simulink model "grua_portuaria"  (R2021a)
settings: Solver=VariableStepAuto  StartTime=0.0  StopTime=2  RelTol=1e-3
values from neighbouring files (symbols this model uses):
  b_cx = 1*10^6    (= 1000000)    [parametros.m]
  b_cy = 1*10^7    (= 10000000)    [parametros.m]
  b_eq = (b_td+b_tm*(r_t^2))/r_td    (= 10803.6)    [parametros.m]
  b_eqh = 2*(b_hd+b_hm*(r_h^2))/r_hd    (= 23253.3333333)    [parametros.m]
  b_ha = b_eqh/r_h - n_h*w_posh*(J_eqh + 0.5*m_l_*r_hd)/r_h    [parametros.m]
  b_hb = 1*10^8    (= 100000000)    [parametros.m]
  b_hEb = 2.2*10^9    (= 2200000000)    [parametros.m]
  b_t = 90    [parametros.m]
  b_ta = n_t*w_post*(r_td*J_eqt/r_t) - r_td*b_eqt/r_t    [parametros.m]
  b_tb = 5*10^6    (= 5000000)    [parametros.m]
  b_tw = 3*10^3    (= 3000)    [parametros.m]
  b_wu = 150    [parametros.m]
  g = 9.80665    [parametros.m]
  H_c = 2.5    [parametros.m]
  J_eq = (J_td+J_tm_tb*(r_t^2))/r_td    (= 15000)    [parametros.m]
  J_eqh = 2*(J_hd_hEb+J_hm_hb*(r_h^2))/r_hd    (= 48853.3333333)    [parametros.m]
  K_cy = 1.8*10^9    (= 1800000000)    [parametros.m]
  K_hsa = -n_h*(w_posh^2)*(J_eqh + 0.5*m_l_*r_hd)/r_t    [parametros.m]
  K_hsia = -(w_posh^3)*(J_eqh + 0.5*m_l_*r_hd)/r_t    [parametros.m]
  K_tsa = n_t*(w_post^2)*J_eqt*r_td/r_t    [parametros.m]
  K_tsia = (w_post^3)*J_eqt*r_td/r_t    [parametros.m]
  K_tw = 4.8*10^5    (= 480000)    [parametros.m]
  k_wu = 2.36*10^8    (= 236000000)    [parametros.m]
  M_s = 15000    [parametros.m]
  M_t = 30000    [parametros.m]
  r_h = 22    [parametros.m]
  r_hd = 0.75    [parametros.m]
  r_t = 30    [parametros.m]
  r_td = 0.5    [parametros.m]
  T_hb_MAX = 5*10^5    (= 500000)    [parametros.m]
  T_hEb_MAX = 1.1*10^6    (= 1100000)    [parametros.m]
  T_s2 = 5e-3    (= 0.005)    [parametros.m]
  T_tb_MAX = 5*10^4    (= 50000)    [parametros.m]
  tau_hm = 1e-3    (= 0.001)    [parametros.m]
  tau_tm = 1e-3    (= 0.001)    [parametros.m]
  Y_t0 = 45    [parametros.m]
undefined symbols (not defined in the file or in its folder): T_s
libraries: simulink x9, dspstat3 x1, vrlib x1
(part 2 of 3)

== stateflow chart grua_portuaria/Nivel 1: Control Supervisor Global/Chart ==
  note: LA VARUABLE Modo_Manual, es la misma que Cambiar_Modo ?
  note: ---> FINES DE CARRERA:
      |
      | 1. FIN DE CARRERA CARRO:
  state Apagado_OFF_
  note: ---> Si el Nivel 1 se encuentra apagodo deberia actuar el Nivel 0
  note: VERIFICAR SI EN VEZ DE PONER == 0 EN UNA CONDICIÓN SE PUEDE PONER COMO BOOL Y SE SIMPLIFICAN MUCHO LAS CONDICIONES.
      | TIPO: ~TLK (TLK ==0) O TLK (TLK == 1)
  note: ---> Activado = Freno Energizado = Freno ABIERTO
  note: ---> Desactivado = Freno NO Energizado = Freno CERRADO
  state Encendido_ON_
    state Fines_de_Carrera [parallel]
      settings: executionOrder=1
      state FIN_DE_CARRERA_CARRO [parallel]
        settings: executionOrder=1
        state Detener_Frenar
          entry:
          Modo_Manual = 1;
          Detener_Carro = 1;
        state Movimiento
          entry:
          Detener_Carro = 0;
        (default) -> Encendido_ON_.Fines_de_Carrera.FIN_DE_CARRERA_CARRO.Movimiento
        Encendido_ON_.Fines_de_Carrera.FIN_DE_CARRERA_CARRO.Detener_Frenar -> Encendido_ON_.Fines_de_Carrera.FIN_DE_CARRERA_CARRO.Movimiento : [(dx_t_ref < 0 && Fin_Der_Lim >= 1) || ((dx_t_ref > 0 && Fin_Izq_Lim >= 1))]
        Encendido_ON_.Fines_de_Carrera.FIN_DE_CARRERA_CARRO.Movimiento -> Encendido_ON_.Fines_de_Carrera.FIN_DE_CARRERA_CARRO.Detener_Frenar : [(Fin_Der_Lim >= 1 && dx_t_ref > 0) || (Fin_Izq_Lim >= 1 && dx_t_ref < 0)]
      state FIN_DE_CARRERA_IZAJE [parallel]
        settings: executionOrder=2
        state Detener_Frenar
          entry:
          Modo_Manual = 1;
          Detener_Izaje = 1;
        state Movimiento
          entry:
          Detener_Izaje = 0;
        (default) -> Encendido_ON_.Fines_de_Carrera.FIN_DE_CARRERA_IZAJE.Movimiento
        Encendido_ON_.Fines_de_Carrera.FIN_DE_CARRERA_IZAJE.Detener_Frenar -> Encendido_ON_.Fines_de_Carrera.FIN_DE_CARRERA_IZAJE.Movimiento : [(dl_h_ref < 0 && Fin_Sup_Lim >= 1) || ((dl_h_ref > 0 && Fin_Inf_Lim >= 1))]
        Encendido_ON_.Fines_de_Carrera.FIN_DE_CARRERA_IZAJE.Movimiento -> Encendido_ON_.Fines_de_Carrera.FIN_DE_CARRERA_IZAJE.Detener_Frenar : [(Fin_Sup_Lim >= 1 && dl_h_ref > 0) || (Fin_Inf_Lim >= 1 && dl_h_ref < 0)]
    state Frenos [parallel]
      settings: executionOrder=2
      note: % Freno desactivado = Frenando
      state FRENO_CARRO [parallel]
        settings: executionOrder=1
        state Desactivado
          entry:
          BRK_t = 0;
          Detener_Carro = 1;
        state Activado
          entry:
          BRK_t = 1;
          Detener_Carro = 0;
        (default) -> Encendido_ON_.Frenos.FRENO_CARRO.Desactivado
        Encendido_ON_.Frenos.FRENO_CARRO.Activado -> Encendido_ON_.Frenos.FRENO_CARRO.Desactivado : [(abs(w_tm) < w_tm_min && dx_t_ref_man == 0) || Falla >0]
        Encendido_ON_.Frenos.FRENO_CARRO.Desactivado -> Encendido_ON_.Frenos.FRENO_CARRO.Activado : [(Freno_Carro_Man == 1) && Falla == 0]
      state FRENO_IZAJE [parallel]
        settings: executionOrder=2
        state Desactivado
          entry:
          BRK_h = 0;
          Detener_Izaje = 1;
        state Activado
          entry:
          BRK_h = 1;
          Detener_Izaje = 0;
        (default) -> Encendido_ON_.Frenos.FRENO_IZAJE.Desactivado
        Encendido_ON_.Frenos.FRENO_IZAJE.Activado -> Encendido_ON_.Frenos.FRENO_IZAJE.Desactivado : [(abs(w_hm) < w_hm_min && dl_h_ref_man == 0) || Falla >0]
        Encendido_ON_.Frenos.FRENO_IZAJE.Desactivado -> Encendido_ON_.Frenos.FRENO_IZAJE.Activado : [(Freno_Izaje_Man == 1) && Falla == 0]
      state FRENO_EMERGENCIA [parallel]
        settings: executionOrder=3
        state Activado
          entry:
          BRK_hE = 1;
        state Desactivado
          entry:
          BRK_hE = 0;
        (default) -> Encendido_ON_.Frenos.FRENO_EMERGENCIA.Desactivado
        Encendido_ON_.Frenos.FRENO_EMERGENCIA.Activado -> Encendido_ON_.Frenos.FRENO_EMERGENCIA.Desactivado : [Grua_Encendida == 0 || Falla > 0]
        Encendido_ON_.Frenos.FRENO_EMERGENCIA.Desactivado -> Encendido_ON_.Frenos.FRENO_EMERGENCIA.Activado : [Grua_Encendida == 1 && Falla == 0]
    state OBSTACULOS [parallel]
      entry:
      [contenedor_posiciones, y_sup] = generar_obstaculos()
      settings: executionOrder=9
      state ACTUALIZACION_CONTENEDORES [parallel]
        settings: executionOrder=1
        state Verificar
        state Cargado
          entry:
          y_l = obtener_posicion_y(y_l, TLK);
          contenedor_posiciones = actualizar_contenedores(contenedor_posiciones, x_td, y_l)
        (default) -> Verificar
        Verificar -> Cargado : [Cable_Tenso == 0 &&  Activar_TLK == 1 && TLK == 0 ]
        Cargado -> Verificar : [Cable_Tenso == 1]
    state Deteccion_Cable_Flojo [parallel]
      settings: executionOrder=3
      state CABLE_FLOJO
        entry:
        Cable_Tenso = 0;
      state CABLE_TENSO
        entry:
        Cable_Tenso = 1;
      (default) -> CABLE_TENSO
      CABLE_FLOJO -> CABLE_TENSO : [F_hw >= Tension_Minima_Cable_Izaje]
      CABLE_TENSO -> CABLE_FLOJO : [F_hw <= Tension_Minima_Cable_Izaje]
    state Senal_De_Vida [parallel]
      settings: executionOrder=4
      state ENVIAR_PULSO
        entry:
        Vida = 1;
      state ESPERA
        entry:
        Vida = 0;
      (default) -> ESPERA
      ENVIAR_PULSO -> ESPERA : [after(50, msec)]
      ESPERA -> ENVIAR_PULSO : [after(450, msec)]
    state Control_De_Balanceo [parallel]
      settings: executionOrder=5
      state ACTIVADO
        entry:
        BAC = 1;
      state DESACTIVADO
        entry:
        BAC = 0;
      (default) -> DESACTIVADO
      ACTIVADO -> DESACTIVADO : [Balanceo == 0 || Falla >0]
      DESACTIVADO -> ACTIVADO : [Balanceo == 1 && Falla == 0]
    state Modo [parallel]
      settings: executionOrder=10
      state MANUAL
        entry:
        Modo_Manual = 1;
        state Carro [parallel]
          settings: executionOrder=1
          state Operacion_Normal
            during:
            dx_t_ref = calcular_velocidad_maximaC(dx_t_SobreV);
          state sobrecarga_Carro
            entry:
            dx_t_ref = 0;
            calcular_velocidad_maximaC(0);
          state Analisis_FDC_D
            during:
            dx_t_ref = calcular_velocidad_maximaC(dx_t_SobreV*(50-x_td)/10);
          state detener_carro
            entry:
            dx_t_ref = 0;
            calcular_velocidad_maximaC(0);
          state Analisis_FDC_I
            during:
            dx_t_ref = calcular_velocidad_maximaC(dx_t_SobreV*(30+x_td)/10);
          (default) -> Encendido_ON_.Modo.MANUAL.Carro.Operacion_Normal
          Analisis_FDC_D -> Encendido_ON_.Modo.MANUAL.Carro.Operacion_Normal : [Detener_Carro == 1 || dx_t_ref_man < 0]
          Encendido_ON_.Modo.MANUAL.Carro.Operacion_Normal -> sobrecarga_Carro [order 1] : [sobrecarga == 1]
          sobrecarga_Carro -> Encendido_ON_.Modo.MANUAL.Carro.Operacion_Normal : [sobrecarga == 0]
          Encendido_ON_.Modo.MANUAL.Carro.Operacion_Normal -> Analisis_FDC_D [order 3] : [x_td >=40 && dx_t_ref_man > 0 && Detener_Carro == 0]
          Analisis_FDC_I -> Encendido_ON_.Modo.MANUAL.Carro.Operacion_Normal : [Detener_Carro == 1 || dx_t_ref_man > 0]
          Encendido_ON_.Modo.MANUAL.Carro.Operacion_Normal -> detener_carro [order 2] : [Detener_Carro == 1]
          detener_carro -> Encendido_ON_.Modo.MANUAL.Carro.Operacion_Normal : [Detener_Carro == 0]
          Encendido_ON_.Modo.MANUAL.Carro.Operacion_Normal -> Analisis_FDC_I [order 4] : [x_td <=-20 && dx_t_ref_man < 0 && Detener_Carro == 0]
        state Izaje [parallel]
          settings: executionOrder=2
          note: dl_h_ref_man se refiere a longitud del cable. Si es >0, se tiene mayor longitud de cable y la carga baja. Si es <0 la longitud disminuye y la carga baja. El 5 en FDC_ARRIBA es una medida de seguridad. En estimacion de masa se limita la velocidad al 10%.
          state Operacion_Normal
            during:
            dl_h_ref = calcular_velocidad_maxima_I(dl_h_SobreV, CT);
          state sobrecarga_Izaje
            during:
            if (dl_h_ref_man>0)
            dl_h_ref = calcular_velocidad_maxima_I(dl_h_SobreV, MasaFija)*0.1;
            else
            dx_t_ref = 0;
            calcular_velocidad_maxima_I(0);
            end
          state Analisis_FDC_ARRIBA
            during:
            dl_h_ref = calcular_velocidad_maxima_I(dl_h_SobreV*(l_h-5)/5, MasaFija);
          state Analisis_FDC_ABAJO
            during:
            dl_h_ref = calcular_velocidad_maxima_I(dl_h_SobreV*(65-l_h)/10, MasaFija);
          state detener_Izaje
            entry:
            dx_t_ref = 0;
            calcular_velocidad_maxima_I(0)
          state Analisis_ESTIMACION_MASA
            during:
            dl_h_ref = calcular_velocidad_maxima_I(dl_h_SobreV, MasaFija)*0.1;
          (default) -> Encendido_ON_.Modo.MANUAL.Izaje.Operacion_Normal
          Analisis_FDC_ARRIBA -> Encendido_ON_.Modo.MANUAL.Izaje.Operacion_Normal : [Detener_Izaje == 1 || dl_h_ref_man > 0]
          Encendido_ON_.Modo.MANUAL.Izaje.Operacion_Normal -> sobrecarga_Izaje [order 1] : [sobrecarga == 1]
          sobrecarga_Izaje -> Encendido_ON_.Modo.MANUAL.Izaje.Operacion_Normal : [sobrecarga == 0]
          Encendido_ON_.Modo.MANUAL.Izaje.Operacion_Normal -> Analisis_FDC_ARRIBA [order 3] : [l_h <=10 && dl_h_ref_man < 0 && Detener_Izaje == 0]
          Analisis_FDC_ABAJO -> Encendido_ON_.Modo.MANUAL.Izaje.Operacion_Normal : [Detener_Izaje == 1 || dl_h_ref_man < 0]
          Encendido_ON_.Modo.MANUAL.Izaje.Operacion_Normal -> Analisis_FDC_ABAJO [order 4] : [l_h <=55 && dl_h_ref_man > 0 && Detener_Izaje == 0]
          Analisis_ESTIMACION_MASA -> Encendido_ON_.Modo.MANUAL.Izaje.Operacion_Normal : [MasaFija == 1 || sobrecarga == 1]
          Encendido_ON_.Modo.MANUAL.Izaje.Operacion_Normal -> detener_Izaje [order 2] : [Detener_Izaje == 1]
          detener_Izaje -> Encendido_ON_.Modo.MANUAL.Izaje.Operacion_Normal : [Detener_Izaje == 0]
          Encendido_ON_.Modo.MANUAL.Izaje.Operacion_Normal -> Analisis_ESTIMACION_MASA [order 5] : [MasaFija == 0 && TLK == 1]
      state AUTOMATICO
        entry:
        Modo_Manual = 0;
        punto_limite = [0, 10];
        punto_muelle = [-20, 4.5];
        y_l = obtener_posicion_y(y_l, TLK);
        punto_inicial = [x_td, y_l];
        if TLK == 1 && Cable_Tenso == 1
        [trayectoria_x, trayectoria_y] = generar_trayectoria_vuelta(y_sup, punto_limite, punto_inicial, punto_muelle);
        else
        posicion_final = obtener_posicion_final(contenedor_posiciones)
        [trayectoria_x, trayectoria_y] = generar_trayectoria_ida(y_sup, punto_limite, punto_inicial, posicion_final);
        end
        % Esto no estoy seguro pero es lo que se me ocurrió quizás habría que calcularlo
        % a partir del tiempo que simulink recorre el ciclo, o pensar algo de no poner puntos de discretizacion
        cant_puntos_discretizacion = 5000;
        perfil_vel_x = obtener_perfil_velocidad('carro', trayectoria_x, TLK, cant_puntos_discretizacion);
        perfil_vel_y = obtener_perfil_velocidad('izaje', trayectoria_y, TLK, cant_puntos_discretizacion);
        perfil_vel_x = perfil_vel_x(:,2)';
        perfil_vel_y = perfil_vel_x(:,2)';
        it = 1;
        during:
        dx_t_ref = perfil_vel_x(it);
        dl_h_ref = perfil_vel_y(it);
        it = it + 1;
        if (it == cant_puntos_discretizacion)
        Cambiar_Modo = 0;
        Modo_Manual = 1;
        end
      note: No entiendo estas condiciones de distinto de 0, por que cambiarían al modo manual ?
      (default) -> MANUAL
      MANUAL -> AUTOMATICO : [Cambiar_Modo == 1]
      AUTOMATICO -> MANUAL [order 1] : [Fin_Der_Lim || Fin_Izq_Lim ]
      AUTOMATICO -> MANUAL [order 2] : [Fin_Sup_Lim || Fin_Inf_Lim]
      AUTOMATICO -> MANUAL [order 3] : [dx_t_ref_man ~= 0]
      AUTOMATICO -> MANUAL [order 4] : [dl_h_ref_man ~= 0]
      AUTOMATICO -> MANUAL [order 5] : [Cambiar_Modo == 0]
    state Sobrevelocidad [parallel]
      settings: executionOrder=7
      note: LA IDEA ES QUE SOLO SE ANALICE LA SOBREVELOCIDAD UNA VEZ QUE LA MASA FUE ESTIMADA, YA QUE ANTES DE ESO SE ELEVA A UNA VELOCIDAD REDUCIDA
      state ANALISI_SOBREVELOCIDAD
        state CARRO [parallel]
          settings: executionOrder=2
          state Analisis_Sobrevelocidad
            entry:
            if (dx_t_ref_man>0)
            dx_t_SobreV = v_t_MAX;
            else
            dx_t_SobreV = v_t_MIN;
            end
          state Actualizacion_Vel_CARRO
            during:
            dx_t_SobreV = dx_t_ref_man
          (default) -> Actualizacion_Vel_CARRO
          Actualizacion_Vel_CARRO -> Analisis_Sobrevelocidad : [abs(dx_t_ref_man) > v_t_MAX]
          Analisis_Sobrevelocidad -> Actualizacion_Vel_CARRO : [abs(dx_t_ref_man) <= v_t_MAX]
        state IZAJE [parallel]
          settings: executionOrder=1
          state Actualizacion_Vel_IZAJE
            during:
            dl_h_SobreV = dl_h_ref_man
          state Analisis_Sobrevelocidad_Pos
            entry:
            dl_h_SobreV = v_t_MAXMIN;
          state Analisis_Sobrevelocidad_Neg
            entry:
            dl_h_SobreV = -v_t_MAXMIN;
          (default) -> Actualizacion_Vel_IZAJE
          Actualizacion_Vel_IZAJE -> Analisis_Sobrevelocidad_Pos [order 1] : [(dl_h_ref_man > v_t_MAXMIN) ]
          Analisis_Sobrevelocidad_Pos -> Actualizacion_Vel_IZAJE : [(dl_h_ref_man <= v_t_MAXMIN) ]
          Actualizacion_Vel_IZAJE -> Analisis_Sobrevelocidad_Neg [order 2] : [(dl_h_ref_man < -v_t_MAXMIN)]
          Analisis_Sobrevelocidad_Neg -> Actualizacion_Vel_IZAJE : [(dl_h_ref_man >= -v_t_MAXMIN)]
      state NO_ANALISIS
      note: EN MODO AUTOMATICO NO DEBERIA SOBREPASARSE LA VELOCIDAD.
      (default) -> NO_ANALISIS
      NO_ANALISIS -> ANALISI_SOBREVELOCIDAD : [MasaFija == 1 ]
      ANALISI_SOBREVELOCIDAD -> NO_ANALISIS : [MasaFija == 0]
    state Sobrecarga [parallel]
      settings: executionOrder=8
      note: SI HAY SOBRECARGA SOLO SE PUEDE BAJAR MANUALMENTE
      state CON_SOBRECARGA
        entry:
        sobrecarga = 1;
        BRK_t = 0;
        BRK_h = 0;
      state SIN_SOBRECARGA1
        entry:
        sobrecarga = 0;
        BRK_t = 1;
        BRK_h = 1;
      state BAJAR_CARGA
        entry:
        BRK_t = 1;
        BRK_h = 1;
      SIN_SOBRECARGA1 -> CON_SOBRECARGA : [M_cX > M_cmax && MasaFija == 1]
      BAJAR_CARGA -> CON_SOBRECARGA [order 1] : [dl_h_ref_man<0]
      BAJAR_CARGA -> SIN_SOBRECARGA1 [order 2] : [Cable_Tenso==0]
      CON_SOBRECARGA -> BAJAR_CARGA : [dl_h_ref_man>0]
      (default) -> SIN_SOBRECARGA1
    state Twistlocks [parallel]
      settings: executionOrder=6
      note: SE ACTIVA EL TLK SI EL OPERARIO LO DESEA Y
          | ADEMAS LA TENSION EN EL CABLE ES 0 (spreader apoyado)
      state TLK_ABIERTO
        entry:
        TLK = 0;
      state TLK_CERRADO
        entry:
        TLK = 1;
      (default) -> TLK_ABIERTO
      TLK_CERRADO -> TLK_ABIERTO : [S_TLK == 1 && Activar_TLK == 0 && Cable_Tenso == 0 && TLK == 1]
      TLK_ABIERTO -> TLK_CERRADO : [S_TLK == 1 &&  Activar_TLK == 1 && Cable_Tenso == 0 && TLK == 0]
  note: Quizás los obstáculos habría que generarlos fuera y enviarlos porque si se llega a apagar el modo automático va a ingresar de nuevo. Pero la lógica es parecida.
      | ???????
  note: Por ahora solo admite ir a buscar los contenedores al barco e ir a dejarlos al muelle. Probemos eso y despues le agregamos los otros modos ( cargar el barco y descargar el barco + buscar contenedor y cargarlo de nuevo)
  Apagado_OFF_ -> Encendido_ON_ : [Alimentacion == 1]
  Encendido_ON_ -> Apagado_OFF_ : [Alimentacion == 0]
  (default) -> Encendido_ON_
  data: dx_manual function_input; v_max_carro function_output; dh_manual function_input; v_max_izaje function_output; Enclave function_input; contenedor_posiciones function_output; y_sup function_output; contenedor_posiciones function_output; contenedor_posiciones function_input; pos_x function_input; pos_y function_input; posicion_final function_output unknown; contenedor_posiciones function_input; l_h function_input; TLK function_input; pos_y_ function_output; y_sup function_input; punto_limite function_input; punto_inicial function_input; punto_final function_input; trayectoria_x function_output; trayectoria_y function_output; y_sup function_input; punto_limite function_input; punto_inicial function_input; punto_final function_input; trayectoria_x function_output; trayectoria_y function_output; tipo function_input; puntos function_input; cargado function_input; perfil_vel function_output; cant_puntos_discretizacion function_input; Alimentacion input; Fin_Der_Lim input; Fin_Izq_Lim input; Fin_Sup_Lim input; Fin_Inf_Lim input; data input; BRK_t output; BRK_h output; BRK_hE output; Vida output; Falla input; Grua_Encendida input; dx_t_ref_man input; dl_h_ref_man input; w_tm input; w_hm input; Freno_Carro_Man input; Freno_Izaje_Man input; Balanceo input; x_td input; l_h input; MasaFija input; v_t_MAXMIN input; Activar_TLK input; M_cX input; S_TLK input; dx_t_ref output; dl_h_ref output; BAC output; TLK output; data1 input
  function v_max_carro = calcular_velocidad_maximaC(dx_manual):
    | function v_max_carro = calcular_velocidad_maximaC(dx_manual)
    | 
    | %--------------------------------------------------------------------------%
    | %---------------------Declaracion variables PERSISTENT---------------------% 
    | %--------------------------------------------------------------------------%
    |             % --> Persistent: local variable in a function that retains its 
    |                             % value in memory between calls to the function
    |     persistent dx_t_ref_manual_anterior;
    |     a_max_carro = 1;     % m/s^2 (aceleracion max para el subsistema carro)
    |     dt = 0.02;           % 20 ms (tiempo de muestreo del statechart)
    |     
    | %--------------------------------------------------------------------------%
    | %------------------Inicialización de variables PERSISTENT------------------% 
    | %--------------------------------------------------------------------------%
    | 
    |     if isempty(dx_t_ref_manual_anterior)
    |         dx_t_ref_manual_anterior = 0;
    |     end
    |     
    | %--------------------------------------------------------------------------%
    | %-----------------------------Lógica principal-----------------------------%
    | %--------------------------------------------------------------------------%
    | % La idea es que el sistema siempre vaya a la maxima velocidad que pueda.
    | % Para eso se utiliza la aceleracion maxima para el subsistema carro en
    | % caso de que la velocidad de referencia no sea lo suficientemente grande.
    | % Si la velocidad supera la velocidad maxima, esta se limita al maximo
    | % permitido.
    | 
    |     if abs(dx_manual) >= abs(dx_t_ref_manual_anterior)
    |         if dx_manual > 0                                                    % Aceleracion +
    |             v_max = a_max_carro * dt + dx_t_ref_manual_anterior;
    |             v_max_carro_aux = max(v_max, dx_manual);
    |         else                                                                % Aceleracion -
    |             v_max = -a_max_carro * dt + dx_t_ref_manual_anterior;
    |             v_max_carro_aux = min(v_max, dx_manual);
    |         end
    |     elseif dx_manual < dx_t_ref_manual_anterior                             % Desaceleracion -
    |         v_max = -a_max_carro * dt + dx_t_ref_manual_anterior;
    |         v_max_carro_aux = min(v_max, dx_manual);
    |     else                                                                    % Desaceleracion +
    |         v_max = a_max_carro * dt + dx_t_ref_manual_anterior;
    |         v_max_carro_aux = max(v_max, dx_manual);
    |     end
    |     
    |     if abs(v_max_carro_aux) > 4
    |         if v_max_carro_aux > 0
    |             v_max_carro_aux = 4;
    |         else
    |             v_max_carro_aux = -4;
    |         end
    |     end
    |     v_max_carro = v_max_carro_aux;
    | 
    |     dx_t_ref_manual_anterior = v_max_carro;
    | end
  function v_max_izaje =   calcular_velocidad_maxima_I(dh_manual, Enclave):
    | function v_max_izaje =   calcular_velocidad_maxima_I(dh_manual, Enclave) % CT es Cable Tenso
    | 
    | %--------------------------------------------------------------------------%
    | %---------------------Declaracion variables PERSISTENT---------------------% 
    | %--------------------------------------------------------------------------%
    |             % --> Persistent: local variable in a function that retains its 
    |                             % value in memory between calls to the function
    |     persistent dy_href_manual_ant;
    |     a_max_y = 0.75;  % m/s^2
    |     dt = 0.02;       % 20 ms (tiempo de muestreo del statechart)
    |     
    | %--------------------------------------------------------------------------%
    | %------------------Inicialización de variables PERSISTENT------------------% 
    | %--------------------------------------------------------------------------%
    | 
    |     if isempty(dy_href_manual_ant)
    |         dy_href_manual_ant = 0;
    |     end
    |     
    | %--------------------------------------------------------------------------%
    | %-----------------------------Lógica principal-----------------------------%
    | %--------------------------------------------------------------------------%
    | % La idea es que el sistema siempre vaya a la maxima velocidad que pueda.
    | % Para eso se utiliza la aceleracion maxima para el subsistema carro en
    | % caso de que la velocidad de referencia no sea lo suficientemente grande.
    | % Si la velocidad supera la velocidad maxima, esta se limita al maximo
    | % permitido.
    | 
    |     if abs(dy_manual) >= abs(dy_href_manual_ant)
    |         if dy_manual > 0
    |             v_max = a_max_y * dt + dy_href_manual_ant;
    |             v_max_izaje_aux = max(v_max, dh_manual);
    |         else
    |             v_max = -a_max_y * dt + dy_href_manual_ant;
    |             v_max_izaje_aux = min(v_max, dh_manual);
    |         end
    |     else
    |         if dy_manual < dy_href_manual_ant
    |             v_max = -a_max_y * dt + dy_href_manual_ant;
    |             v_max_izaje_aux = min(v_max, dh_manual);
    |         else
    |             v_max = a_max_y * dt + dy_href_manual_ant;
    |             v_max_izaje_aux = max(v_max, dh_manual);
    |         end
    |     end
    |     
    |     if Enclave == 1      % Hay carga, velocidad maxima 1.5 m/s
    |         if abs(v_max_izaje_aux) > 1.5
    |             if v_max_izaje_aux > 0
    |                 v_max_izaje_aux = 1.5;
    |             else
    |                 v_max_izaje_aux = -1.5;
    |             end
    |         end
    |     else                % No hay carga, velocidad maxima 3 m/s
    |         if abs(v_max_izaje_aux) > 3
    |             if v_max_izaje_aux > 0
    |                 v_max_izaje_aux = 3;
    |             else
    |                 v_max_izaje_aux = -3;
    |             end
    |         end
    |     end
    |     v_max_izaje = v_max_izaje_aux;
    |     dy_href_manual_ant = v_max_izaje;
    | 
    | end
  function [contenedor_posiciones, y_sup] = generar_obstaculos:
    | function [contenedor_posiciones, y_sup] = generar_obstaculos()
    |     % Inicializar la figura
    |     figure;
    |     hold on;
    |     xlabel('x');
    |     ylabel('y');
    |     grid on;
    |     axis([-35, 55, -20, 50]);
    | 
    |     % Izaje
    |     hc_izaje = 2.5;
    |     x_izaje = -35:55;
    |     yt0 = ones(size(x_izaje)) * 45;
    |     plot(x_izaje, yt0, '*b');
    | 
    |     % Muelle
    |     % Línea horizontal
    |     x_muelle_h = -35:0;
    |     y_muelle_h = zeros(size(x_muelle_h));
    |     plot(x_muelle_h, y_muelle_h, 'k', 'LineWidth', 2);
    | 
    |     % Línea vertical
    |     y_muelle_v = -20:0;
    |     x_muelle_v = zeros(size(y_muelle_v));
    |     plot(x_muelle_v, y_muelle_v, 'k', 'LineWidth', 2);
    | 
    |     % Barco
    |     % Horizontal abajo
    |     x_barco_h_a = 2.5:50;
    |     y_barco_h_a = ones(size(x_barco_h_a)) * -20;
    |     plot(x_barco_h_a, y_barco_h_a, 'y', 'LineWidth', 4);
    | 
    |     % Horizontal izquierda
    |     x_barco_h_i = 0:2.5;
    |     y_barco_h_i = zeros(size(x_barco_h_i));
    |     plot(x_barco_h_i, y_barco_h_i, 'y', 'LineWidth', 4);
    | 
    |     % Vertical izquierda
    |     y_barco_v = -20:0;
    |     x_barco_v_i = ones(size(y_muelle_v)) * 2.5;
    |     plot(x_barco_v_i, y_barco_v, 'y', 'LineWidth', 4);
    | 
    |     % Vertical derecha
    |     x_barco_v_d = ones(size(y_muelle_v)) * 50;
    |     plot(x_barco_v_d, y_barco_v, 'y', 'LineWidth', 4);
    | 
    |     % Contenedores dentro del barco
    |     num_filas = 16;
    |     num_contenedores_min = 10;
    |     num_contenedores_max = 18;
    | 
    |     % Dibujo de todos los contenedores y perfil de seguridad
    |     for fila = 1:num_filas
    |         % Dibujo de todos los contenedores en la fila actual
    |         num_contenedores_fila = randi([num_contenedores_min, num_contenedores_max]);
    |         posiciones_fila = zeros(num_contenedores_fila, 2);
    | 
    |         for i = 1:num_contenedores_fila
    |             pos_x = 2.5 + (fila - 1) * 3;
    |             pos_y = -20 + (i - 1) * 2.5;
    | 
    |             % Dibuja el contenedor
    |             rectangle('Position', [pos_x, pos_y, 2.5, 2.5], 'EdgeColor', 'r', 'LineWidth', 2);
    | 
    |             % Almacena la posición del contenedor
    |             posiciones_fila(i, :) = [pos_x, pos_y];
    | 
    |             % Etiqueta 'x' en el centro del contenedor
    |             x_center = pos_x + 1.25;
    |             y_center = pos_y + 1.25;
    |             text(x_center, y_center, 'x', 'Color', 'r', 'FontSize', 12, 'HorizontalAlignment', 'center', 'VerticalAlignment', 'middle');
    |         end
    | 
    |         % Almacena las posiciones de la fila
    |         contenedor_posiciones{fila} = posiciones_fila;
    |     end
    |     posiciones = vertcat(contenedor_posiciones{:});
    |     coef_seguridad = 5;
    |     y_sup = max(posiciones(:, 2)) + coef_seguridad;
    | end
  function contenedor_posiciones = actualizar_contenedores(contenedor_posiciones, pos_x, pos_y):
    | function contenedor_posiciones = actualizar_contenedores(contenedor_posiciones, pos_x, pos_y)
    |     for i = 1:size(contenedor_posiciones, 2)
    |         if size(contenedor_posiciones{i},1) ~= 0 % Es decir si quedan contenedores en esa columna
    |             pos_x_inferior_izq_contenedor = contenedor_posiciones{i}(1,1);
    |             pos_x_inferior_der_contenedor = contenedor_posiciones{i}(1,1) + 2.5;
    |             pos_y_sup_contenedor = contenedor_posiciones{i}(end,2) + 2.5;
    |             tolerancia = 0.2;
    |             pos_y_sup_contenedor = pos_y_sup_contenedor + tolerancia;
    |             if pos_x > pos_x_inferior_izq_contenedor && pos_x < pos_x_inferior_der_contenedor && pos_y < pos_y_sup_contenedor 
    |                 contenedor_posiciones{i}(end,:) = []; % Elimino el contenedor de arriba
    |                 break;
    |             end
    |         end
    |     end
    | end
  function posicion_final = obtener_posicion_final(contenedor_posiciones):
    | function posicion_final = obtener_posicion_final(contenedor_posiciones)
    |     posicion_final = [0, 0];
    |     posicion_encontrada = false;
    |     % En principio busca posiciones de izquierda a derecha de los
    |     % contenedores
    |     for i = 1:size(contenedor_posiciones, 2)
    |         if size(contenedor_posiciones{i},1) ~= 0 % Es decir si quedan contenedores en esa columna
    |             fila_final = size(contenedor_posiciones{i}, 1);
    |             posicion_final = contenedor_posiciones{i}(fila_final, :);
    |             % Como tengo la posición del contenedor inferior izquierda le sumo la
    |             % constante para obtener la final
    |             altura_a_manual = 2.5;
    |             cte_contenedor = [1.25, 2.5 + altura_a_manual];
    |             posicion_encontrada = true;
    |             posicion_final = posicion_final + cte_contenedor;
    |             break;
    |         end
    |     end
    |     if ~posicion_encontrada
    |         posicion_final = [-30, 40]; % Lo pongo en la esquina superior izquierda.
    |     end
    | end
  function pos_y_ = obtener_posicion_y(l_h, TLK):
    | function pos_y_ = obtener_posicion_y(l_h, TLK)
    |     if (TLK == 1)
    |         pos_y_=45-l_h-2.5;
    |     else
    |         pos_y_=45-l_h;
    |     end
    | end
  function [trayectoria_x, trayectoria_y] = generar_trayectoria_ida(y_sup, punto_limite, punto_inicial, punto_final):
    | function [trayectoria_x, trayectoria_y] = generar_trayectoria_ida(y_sup, punto_limite, punto_inicial, punto_final)
    |     % Parámetros
    |     grados = 30;
    |     coef_seguridad = 3;
    | 
    |     % Ajustes iniciales
    |     punto_limite(2) = punto_limite(2) + coef_seguridad;
    |     tang = tan(grados*pi/180);
    | 
    |     % Inicializar trayectoria
    |     trayectoria_x = punto_inicial(1);
    |     trayectoria_y = punto_inicial(2);
    |     pos_actual = punto_inicial;
    | 
    |     % Verificar si está cerca del borde del muelle para subir directamente
    |     if pos_actual(1) < -5
    |         % Si la pos_actual es mayor a la y_sup directamente va a avanzar
    |         if pos_actual(2) < y_sup
    |             % Primer tramo (subir línea recta)
    |             altura_subir_bajar = 25;
    |             punto_a_subir = pos_actual(2) + altura_subir_bajar;
    | 
    |             % Verificar si puede hacer un primer tramo en línea recta sin superar la parte superior
    |             if punto_a_subir < y_sup
    |                 pos_actual(2) = punto_a_subir;
    |                 trayectoria_x = [trayectoria_x, pos_actual(1)];
    |                 trayectoria_y = [trayectoria_y, pos_actual(2)];
    |             end
    | 
    |             % Segundo tramo (subir oblicuo)
    |             pos_actual(1) = pos_actual(1) + tang * (y_sup - pos_actual(2));
    |             pos_actual(2) = y_sup;
    |             trayectoria_x = [trayectoria_x, pos_actual(1)];
    |             trayectoria_y = [trayectoria_y, pos_actual(2)];   
    |         end
    | 
    |     else
    |         % Primer tramo (subir/bajar línea recta)
    |         pos_actual(2) = y_sup;
    |         trayectoria_x = [trayectoria_x, pos_actual(1)];
    |         trayectoria_y = [trayectoria_y, pos_actual(2)];
    |     end
    | 
    |     % Tercer y cuarto tramo (avanzar en horizontal y bajar en oblicuo)
    |     puede_bajar = false;
    |     while ~puede_bajar
    |         m = (punto_final(2) - y_sup) / (punto_final(1) - pos_actual(1));
    |         b = pos_actual(2) - m * pos_actual(1);
    | 
    |         interseccion_x = m * punto_limite(1) + b;
    |         interseccion_y = (punto_limite(2) - b) / m;
    | 
    |         if interseccion_x <= punto_limite(2) || interseccion_x <= punto_limite(1)
    |             pos_actual = [pos_actual(1) + 0.5, pos_actual(2)];
    |             trayectoria_x = [trayectoria_x, pos_actual(1)];
    |             trayectoria_y = [trayectoria_y, pos_actual(2)];
    |         else
    |             puede_bajar = true;
    |         end
    |     end
    | 
    |     % Quinto tramo (bajar en línea recta)
    |     trayectoria_x = [trayectoria_x, punto_final(1)];
    |     trayectoria_y = [trayectoria_y, punto_final(2)];
    | end
  function [trayectoria_x, trayectoria_y] = generar_trayectoria_vuelta(y_sup, punto_limite, punto_inicial, punto_final):
    | function [trayectoria_x, trayectoria_y] = generar_trayectoria_vuelta(y_sup, punto_limite, punto_inicial, punto_final)
    |     % Parámetros
    |     grados = 30;
    |     coef_seguridad = 3;
    |     altura_bajar = 25; % Altura desde donde empieza a bajar en línea recta
    | 
    |     % Ajustes iniciales
    |     punto_limite(2) = punto_limite(2) + coef_seguridad;
    |     tang = tan(grados*pi/180);
    | 
    |     % Inicializar trayectoria
    |     trayectoria_x = punto_inicial(1);
    |     trayectoria_y = punto_inicial(2);
    |     pos_actual = punto_inicial;
    | 
    |     % Primer y segundo tramo (subir en línea recta y subir en oblicuo)
    |     puede_subir = false;
    |     while ~puede_subir
    |         dist = tang * (y_sup - pos_actual(2));
    |         m = (y_sup - pos_actual(2)) / ((pos_actual(1) - dist) - pos_actual(1));
    |         b = pos_actual(2) - m * pos_actual(1);
    | 
    |         interseccion_x = m * punto_limite(1) + b;
    |         interseccion_y = (punto_limite(2) - b) / m;
    | 
    |         if interseccion_x <= punto_limite(2) || interseccion_x <= punto_limite(1)
    |             pos_actual = [pos_actual(1), pos_actual(2) + 0.5];
    |             trayectoria_x = [trayectoria_x, pos_actual(1)];
    |             trayectoria_y = [trayectoria_y, pos_actual(2)];
    |         else
    |             puede_subir = true;
    |         end
    |     end
    | 
    |     % Ajuste de posición después de subir en oblicuo
    |     pos_actual(1) = pos_actual(1) - dist;
    |     pos_actual(2) = y_sup;
    |     trayectoria_x = [trayectoria_x, pos_actual(1)];
    |     trayectoria_y = [trayectoria_y, pos_actual(2)];
    | 
    |     % Tercer tramo (línea recta horizontal)
    |     punto_final_linea_recta = [punto_final(1) + tang * (y_sup - altura_bajar), y_sup];
    |     if punto_final_linea_recta(1) < pos_actual(1)
    |         trayectoria_x = [trayectoria_x, punto_final_linea_recta(1)];
    |         trayectoria_y = [trayectoria_y, punto_final_linea_recta(2)];
    |     end
    | 
    |     % Cuarto tramo (bajar en oblicuo)
    |     trayectoria_x = [trayectoria_x, punto_final(1)];
    |     trayectoria_y = [trayectoria_y, punto_final(2) + altura_bajar];
    | 
    |     % Quinto tramo (bajar en línea recta)
    |     trayectoria_x = [trayectoria_x, punto_final(1)];
    |     trayectoria_y = [trayectoria_y, punto_final(2)];
    | end
  function perfil_vel  = obtener_perfil_velocidad(tipo, puntos, cargado, cant_puntos_discretizacion):
    | function perfil_vel  = obtener_perfil_velocidad(tipo, puntos, cargado, cant_puntos_discretizacion)
    |     % Obtener parámetros de aceleración y velocidad máxima
    |     [a_max, v_max] = obtenerParametros(tipo, cargado);
    | 
    |     % Inicializar el perfil de velocidad
    |     perfil_vel = zeros(1, 2);
    |     
    |     % Calcular el tiempo de transición
    |     t_trans = v_max / a_max;
    |     
    |     % Iterar sobre los puntos
    |     t_ant = 0;
    |     for i = 1:numel(puntos)-1
    |         dist = puntos(i+1) - puntos(i);
    |         abs_dist = abs(dist);
    |         
    |         % Calcular tiempo en tramo constante
    |         t_cte = abs_dist / v_max - t_trans;
    |         
    |         if t_cte > 0
    |             % Tramo con velocidad constante
    |             perfil_vel = [perfil_vel; 
    |                 t_ant + t_trans, sign(dist)*v_max; 
    |                 t_ant + t_trans + t_cte, sign(dist)*v_max; 
    |                 t_ant + t_trans*2 + t_cte, 0];
    |         elseif t_cte == 0
    |             % Tramo sin velocidad constante pero llegando a la v_max
    |             perfil_vel = [perfil_vel; 
    |                 t_ant + t_trans, sign(dist)*v_max; 
    |                 t_ant + t_trans*2, 0];
    |         else
    |             % Tramo sin velocidad constante sin llegar a la v_max
    |             v_x = sqrt(a_max*abs_dist);
    |             t_x = abs_dist/v_x;
    |             perfil_vel = [perfil_vel; 
    |                 t_ant + t_x, sign(dist)*v_x; 
    |                 t_ant + t_x*2, 0];
    |         end
    |         
    |         % Actualizar tiempo anterior
    |         t_ant = perfil_vel(end, 1);
    |     end
    |     % Discretizar el perfil de velocidad al final
    |     % La opción 'pchip' en interp1 realiza una interpolación cúbica
    |     t_vals_discretizados = linspace(perfil_vel(1, 1), perfil_vel(end, 1), cant_puntos_discretizacion);
    |     v_vals_discretizados = interp1(perfil_vel(:, 1), perfil_vel(:, 2), t_vals_discretizados, 'pchip');
    |     
    |     perfil_vel = [t_vals_discretizados', v_vals_discretizados'];
    | end
    | 
    | function [a_max, v_max] = obtenerParametros(tipo, cargado)
    |     switch tipo
    |         case 'carro'
    |             a_max = 1;
    |             v_max = 4;
    |         otherwise
    |             a_max = 0.75;
    |             v_max = cargado * 1.5 + ~cargado * 3;
    |     end
    | end

== stateflow chart grua_portuaria/Modelo Físico/TwistLock/Chart ==
  (default) -> (junction 14)
  (junction 14) -> (junction 16) [order 1] : [TLK == 0]
  (junction 14) -> (junction 18) [order 2] : {m_l = M_s + M_Cx; h_c  = H_c}
  (junction 16) -> (junction 20) : {m_l = M_s; h_c =0}
  (junction 20) -> (junction 18)
  (junction 18) -> (junction 23)
  data: TLK input; M_Cx input; m_l output; h_c output; H_c parameter; M_s parameter

== stateflow chart grua_portuaria/Nivel 0: Seguridad o Proteccion/Chart ==
  state Espera
    entry:
    Emergencia = 0;
    BRK_t = 1;
    BRK_h = 1;
    BRK_hE = 1;
    Ciclos = 0;
    state BOTON_EMERGENCIA [parallel]
      settings: executionOrder=1
      state Espera
      state Emergencia
        entry:
        Emergencia = 1;
      (default) -> Espera.BOTON_EMERGENCIA.Espera
      Espera.BOTON_EMERGENCIA.Espera -> Espera.BOTON_EMERGENCIA.Emergencia : [Boton_Emergencia == 1]
    state FINES_DE_CARRERA_AV [parallel]
      settings: executionOrder=2
      state Fin_AV_Carro
        entry:
        Emergencia = 2;
      state Espera
      state Fin_AV_Izaje
        entry:
        Emergencia = 3;
      Espera.FINES_DE_CARRERA_AV.Espera -> Fin_AV_Carro [order 1] : [Fin_Der_Av || Fin_Izq_Av ]
      (default) -> Espera.FINES_DE_CARRERA_AV.Espera
      Espera.FINES_DE_CARRERA_AV.Espera -> Fin_AV_Izaje [order 2] : [Fin_Sup_Av || Fin_Inf_Av ]
    state VIDA_WATCHDOG [parallel]
      settings: executionOrder=3
      state Espera
      state Contador_Ciclos
        entry:
        Ciclos = Ciclos + 1;
      state Hay_Vida
        entry:
        Ciclos = 0;
      state No_Vida
        entry:
        Emergencia = 1;
      (default) -> Espera.VIDA_WATCHDOG.Espera
      Espera.VIDA_WATCHDOG.Espera -> Contador_Ciclos [order 1] : after(550,msec)
      Contador_Ciclos -> Espera.VIDA_WATCHDOG.Espera [order 2]
      Hay_Vida -> Espera.VIDA_WATCHDOG.Espera
      Espera.VIDA_WATCHDOG.Espera -> Hay_Vida [order 2] : [Vida == 1]
      Contador_Ciclos -> No_Vida [order 1] : [Ciclos == 3]
    state SOBREVELOCIDAD [parallel]
      settings: executionOrder=4
      state Emergencia
        entry:
        Emergencia = 2;
      state Espera
      state Emergencia1
        entry:
        Emergencia = 3;
      (default) -> Espera.SOBREVELOCIDAD.Espera
      Espera.SOBREVELOCIDAD.Espera -> Espera.SOBREVELOCIDAD.Emergencia [order 1] : [w_tm > w_tm_max*1.15 ]
      Espera.SOBREVELOCIDAD.Espera -> Emergencia1 [order 2] : [ w_hm > w_hm_max*1.15]
  note: --> El nivel 1 deberia mandar señales de vida
      |      cada 500 msec. Si por más de 3 ciclos no manda señales entra en
      |      modo de emergencia
  state Emergencia_CARRO
    entry:
    BRK_t = 0;
  state Emergencia_TOTAL
    entry:
    BRK_t = 0;
    BRK_h = 0;
    BRK_hE = 0;
  state Emergencia_IZAJE
    entry:
    BRK_h = 0;
    BRK_hE = 0;
  (default) -> Espera
  Espera -> Emergencia_CARRO [order 2] : [Emergencia == 2]
  Emergencia_CARRO -> Espera : [Reinicio == 1]
  Emergencia_TOTAL -> Espera : [Reinicio == 1]
  Espera -> Emergencia_TOTAL [order 1] : [Emergencia == 1]
  Emergencia_IZAJE -> Espera : [Reinicio == 1]
  Espera -> Emergencia_IZAJE [order 3] : [Emergencia == 3]
  data: Boton_Emergencia input; BRK_t output; BRK_h output; BRK_hE output; Reinicio input; Fin_Der_Av input; Fin_Izq_Av input; Fin_Sup_Av input; Fin_Inf_Av input; data input; Emergencia output; v_tm input; v_hm input

== matlab function grua_portuaria/Estimacion de Masa/MATLAB Function ==
  data: tension input; m_l output; M_cX output; TLK input; MasaFija output
function [m_l, M_cX, MasaFija] = fcn(tension, TLK)

%--------------------------------------------------------------------------%
%---------------------Declaracion variables PERSISTENT---------------------% 
%--------------------------------------------------------------------------%
            % --> Persistent: local variable in a function that retains its 
                            % value in memory between calls to the function
    persistent masaPromedio
    persistent contador
    persistent masaEnclavada
    persistent masaFijada
    
    Masa_Spreader = 15000; % Kg
    Peso_Spreader = Masa_Spreader * 9.8;

%--------------------------------------------------------------------------%
%------------------Inicialización de variables PERSISTENT------------------% 
%--------------------------------------------------------------------------%
    if isempty(masaPromedio)
        masaPromedio = zeros(1, 100);
    end
    if isempty(contador)
        contador = 0;
    end
    if isempty(masaEnclavada)
        masaEnclavada = 0;
    end
    if isempty(masaFijada)
        masaFijada = 0;
    end
    
%--------------------------------------------------------------------------%
%-----------------------------Lógica principal-----------------------------%
%--------------------------------------------------------------------------%

    if TLK == 1 && masaEnclavada == 0             % Si la masa ya está enclavada no vuelve a entrar para evitar que variaciones en la tensión afecten
        if tension > Peso_Spreader*1.1            % Peso Spreader + 10%
            m_l = tension * 2 / 9.81;             % El 2 es por la polea
            M_cX = m_l - Masa_Spreader;
            MasaFija = 0;                         % Valor booleano de salida 
            contador = contador + 1;
 
            if contador > length(masaPromedio)    % Por lo menos 100 masas para calcular el promedio
                masaPromedio = masaPromedio(2:end);
                masaPromedio = [masaPromedio, m_l];
                promedio = sum(masaPromedio) / length(masaPromedio);

                if promedio < (m_l + 1000) && promedio > (m_l - 1000)
                    masaEnclavada = 1;
                    masaFijada = m_l;
                    MasaFija = 1;
                end
            else
                masaPromedio(contador) = m_l;
            end
        else
            m_l = 41000;                    % Valor inicial de masa (Promedio entre Max y Min + Spreader)
            M_cX = m_l - Masa_Spreader;
            MasaFija = 0;
        end
    elseif TLK == 0
        masaEnclavada = 0;
        contador = 0;
        m_l = Masa_Spreader ;
        M_cX = m_l - Masa_Spreader;
        MasaFija = 0;
    elseif masaEnclavada == 1
        m_l = masaFijada;
        M_cX = m_l - Masa_Spreader;
        MasaFija = 1;
    end
end

== matlab function grua_portuaria/MATLAB Function ==
  data: masa input; velocidad_maxima output
function velocidad_maxima = calcular_velocidad_maxima_Izaje(masa)
    % Puntos conocidos (masa, velocidad)
    puntos_conocidos = [
        65000, 1.5;
        60000, 1.67;
        53000, 1.83;
        50000, 1.9;
        48000, 2;
        45000, 2.1;
        44000, 2.166;
        41000, 2.33;
        40000, 2.4;
        38000, 2.5;
        35000, 2.7;
        34000, 2.88;
        32000, 3;
        30000, 3;
        25000, 3;
        20000, 3;
        15000, 3
    ];

    % Realizar interpolación lineal
    velocidad_maxima = interp1(puntos_conocidos(:, 1), puntos_conocidos(:, 2), masa, 'linear');

    % Asegurarse de que la velocidad no sea NaN si la masa está fuera del rango
    if isnan(velocidad_maxima)
        velocidad_maxima = 0;
    end
end

== stateflow chart grua_portuaria/JOYSTICK/Mantener Seleccion ==
  state Espera
  state Invertir
    entry:
    X_=(~X_);
  (default) -> Espera
  Espera -> Invertir : [X~=0]
  Invertir -> Espera : [X==0]
  data: X input; X_ output boolean =false

== stateflow chart grua_portuaria/JOYSTICK/Mantener Seleccion2 ==
  state Espera
  state Invertir
    entry:
    a_=(~a_);
  (default) -> Espera
  Espera -> Invertir : [a~=0]
  Invertir -> Espera : [a==0]
  data: a input; a_ output boolean =false
